simulink model "BMS_Software_NXP_Rolo"  (R2020a)
settings: Solver=FixedStepDiscrete  StartTime=0.0  StopTime=10.0  FixedStep=0.05  RelTol=1e-3  EnableMultiTasking=on
InitFcn:
  | mbd_s32k_consistency_checks(bdroot(gcs));
undefined symbols (not defined in the file or in its folder): LQFP
libraries: mbd_bcc_ec_toolbox x51, mbd_s32k1xx_ec_toolbox x16
(part 2 of 3)

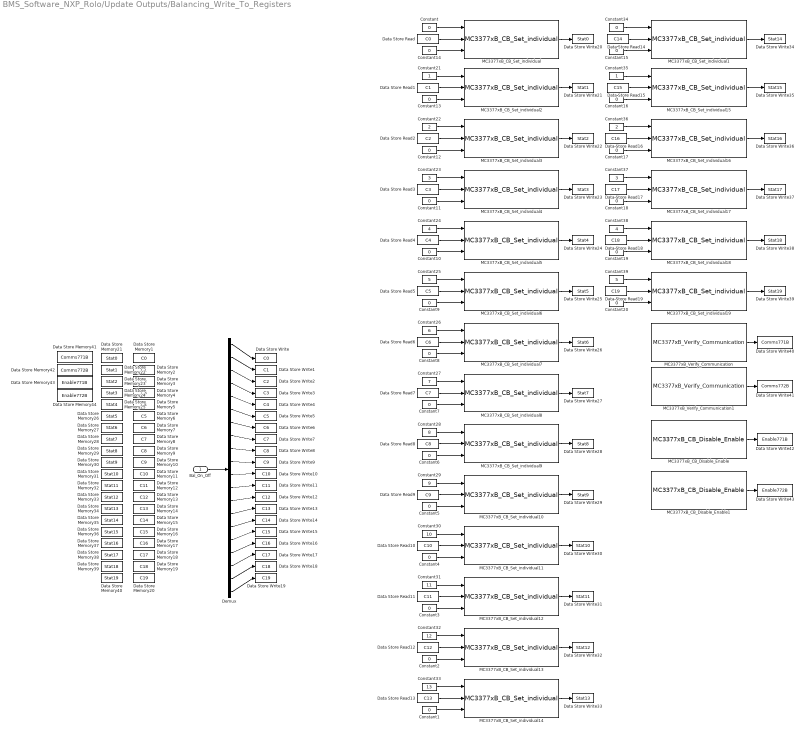
== system BMS_Software_NXP_Rolo/Update Outputs/Balancing_Write_To_Registers ==
  Bal_On_Off : Inport
  Constant : Constant  Value=0  OutDataTypeStr=uint8
  Constant{1..20} (20 alike) : Constant  Value=0  OutDataTypeStr=uint16
  Constant21 : Constant  OutDataTypeStr=uint8
  Constant22 : Constant  Value=2  OutDataTypeStr=uint8
  Constant23 : Constant  Value=3  OutDataTypeStr=uint8
  Constant24 : Constant  Value=4  OutDataTypeStr=uint8
  Constant25 : Constant  Value=5  OutDataTypeStr=uint8
  Constant26 : Constant  Value=6  OutDataTypeStr=uint8
  Constant27 : Constant  Value=7  OutDataTypeStr=uint8
  Constant28 : Constant  Value=8  OutDataTypeStr=uint8
  Constant29 : Constant  Value=9  OutDataTypeStr=uint8
  Constant30 : Constant  Value=10  OutDataTypeStr=uint8
  Constant31 : Constant  Value=11  OutDataTypeStr=uint8
  Constant32 : Constant  Value=12  OutDataTypeStr=uint8
  Constant33 : Constant  Value=13  OutDataTypeStr=uint8
  Constant34 : Constant  Value=0  OutDataTypeStr=uint8
  Constant35 : Constant  OutDataTypeStr=uint8
  Constant36 : Constant  Value=2  OutDataTypeStr=uint8
  Constant37 : Constant  Value=3  OutDataTypeStr=uint8
  Constant38 : Constant  Value=4  OutDataTypeStr=uint8
  Constant39 : Constant  Value=5  OutDataTypeStr=uint8
  Data Store Memory1 : DataStoreMemory  DataStoreName=C0  ReadBeforeWriteMsg=warning  WriteAfterWriteMsg=warning  WriteAfterReadMsg=warning  ShowAdditionalParam=off  OutDataTypeStr=boolean
  Data Store Memory10 : DataStoreMemory  DataStoreName=C9  ReadBeforeWriteMsg=warning  WriteAfterWriteMsg=warning  WriteAfterReadMsg=warning  ShowAdditionalParam=off  OutDataTypeStr=boolean
  Data Store Memory11 : DataStoreMemory  DataStoreName=C10  ReadBeforeWriteMsg=warning  WriteAfterWriteMsg=warning  WriteAfterReadMsg=warning  ShowAdditionalParam=off  OutDataTypeStr=boolean
  Data Store Memory12 : DataStoreMemory  DataStoreName=C11  ReadBeforeWriteMsg=warning  WriteAfterWriteMsg=warning  WriteAfterReadMsg=warning  ShowAdditionalParam=off  OutDataTypeStr=boolean
  Data Store Memory13 : DataStoreMemory  DataStoreName=C12  ReadBeforeWriteMsg=warning  WriteAfterWriteMsg=warning  WriteAfterReadMsg=warning  ShowAdditionalParam=off  OutDataTypeStr=boolean
  Data Store Memory14 : DataStoreMemory  DataStoreName=C13  ReadBeforeWriteMsg=warning  WriteAfterWriteMsg=warning  WriteAfterReadMsg=warning  ShowAdditionalParam=off  OutDataTypeStr=boolean
  Data Store Memory15 : DataStoreMemory  DataStoreName=C14  ReadBeforeWriteMsg=warning  WriteAfterWriteMsg=warning  WriteAfterReadMsg=warning  ShowAdditionalParam=off  OutDataTypeStr=boolean
  Data Store Memory16 : DataStoreMemory  DataStoreName=C15  ReadBeforeWriteMsg=warning  WriteAfterWriteMsg=warning  WriteAfterReadMsg=warning  ShowAdditionalParam=off  OutDataTypeStr=boolean
  Data Store Memory17 : DataStoreMemory  DataStoreName=C16  ReadBeforeWriteMsg=warning  WriteAfterWriteMsg=warning  WriteAfterReadMsg=warning  ShowAdditionalParam=off  OutDataTypeStr=boolean
  Data Store Memory18 : DataStoreMemory  DataStoreName=C17  ReadBeforeWriteMsg=warning  WriteAfterWriteMsg=warning  WriteAfterReadMsg=warning  ShowAdditionalParam=off  OutDataTypeStr=boolean
  Data Store Memory19 : DataStoreMemory  DataStoreName=C18  ReadBeforeWriteMsg=warning  WriteAfterWriteMsg=warning  WriteAfterReadMsg=warning  ShowAdditionalParam=off  OutDataTypeStr=boolean
  Data Store Memory2 : DataStoreMemory  DataStoreName=C1  ReadBeforeWriteMsg=warning  WriteAfterWriteMsg=warning  WriteAfterReadMsg=warning  ShowAdditionalParam=off  OutDataTypeStr=boolean
  Data Store Memory20 : DataStoreMemory  DataStoreName=C19  ReadBeforeWriteMsg=warning  WriteAfterWriteMsg=warning  WriteAfterReadMsg=warning  ShowAdditionalParam=off  OutDataTypeStr=boolean
  Data Store Memory21 : DataStoreMemory  DataStoreName=Stat0  ReadBeforeWriteMsg=warning  WriteAfterWriteMsg=warning  WriteAfterReadMsg=warning  ShowAdditionalParam=off  OutDataTypeStr=uint8
  Data Store Memory22 : DataStoreMemory  DataStoreName=Stat1  ReadBeforeWriteMsg=warning  WriteAfterWriteMsg=warning  WriteAfterReadMsg=warning  ShowAdditionalParam=off  OutDataTypeStr=uint8
  Data Store Memory23 : DataStoreMemory  DataStoreName=Stat2  ReadBeforeWriteMsg=warning  WriteAfterWriteMsg=warning  WriteAfterReadMsg=warning  ShowAdditionalParam=off  OutDataTypeStr=uint8
  Data Store Memory24 : DataStoreMemory  DataStoreName=Stat3  ReadBeforeWriteMsg=warning  WriteAfterWriteMsg=warning  WriteAfterReadMsg=warning  ShowAdditionalParam=off  OutDataTypeStr=uint8
  Data Store Memory25 : DataStoreMemory  DataStoreName=Stat4  ReadBeforeWriteMsg=warning  WriteAfterWriteMsg=warning  WriteAfterReadMsg=warning  ShowAdditionalParam=off  OutDataTypeStr=uint8
  Data Store Memory26 : DataStoreMemory  DataStoreName=Stat5  ReadBeforeWriteMsg=warning  WriteAfterWriteMsg=warning  WriteAfterReadMsg=warning  ShowAdditionalParam=off  OutDataTypeStr=uint8
  Data Store Memory27 : DataStoreMemory  DataStoreName=Stat6  ReadBeforeWriteMsg=warning  WriteAfterWriteMsg=warning  WriteAfterReadMsg=warning  ShowAdditionalParam=off  OutDataTypeStr=uint8
  Data Store Memory28 : DataStoreMemory  DataStoreName=Stat7  ReadBeforeWriteMsg=warning  WriteAfterWriteMsg=warning  WriteAfterReadMsg=warning  ShowAdditionalParam=off  OutDataTypeStr=uint8
  Data Store Memory29 : DataStoreMemory  DataStoreName=Stat8  ReadBeforeWriteMsg=warning  WriteAfterWriteMsg=warning  WriteAfterReadMsg=warning  ShowAdditionalParam=off  OutDataTypeStr=uint8
  Data Store Memory3 : DataStoreMemory  DataStoreName=C2  ReadBeforeWriteMsg=warning  WriteAfterWriteMsg=warning  WriteAfterReadMsg=warning  ShowAdditionalParam=off  OutDataTypeStr=boolean
  Data Store Memory30 : DataStoreMemory  DataStoreName=Stat9  ReadBeforeWriteMsg=warning  WriteAfterWriteMsg=warning  WriteAfterReadMsg=warning  ShowAdditionalParam=off  OutDataTypeStr=uint8
  Data Store Memory31 : DataStoreMemory  DataStoreName=Stat10  ReadBeforeWriteMsg=warning  WriteAfterWriteMsg=warning  WriteAfterReadMsg=warning  ShowAdditionalParam=off  OutDataTypeStr=uint8
  Data Store Memory32 : DataStoreMemory  DataStoreName=Stat11  ReadBeforeWriteMsg=warning  WriteAfterWriteMsg=warning  WriteAfterReadMsg=warning  ShowAdditionalParam=off  OutDataTypeStr=uint8
  Data Store Memory33 : DataStoreMemory  DataStoreName=Stat12  ReadBeforeWriteMsg=warning  WriteAfterWriteMsg=warning  WriteAfterReadMsg=warning  ShowAdditionalParam=off  OutDataTypeStr=uint8
  Data Store Memory34 : DataStoreMemory  DataStoreName=Stat13  ReadBeforeWriteMsg=warning  WriteAfterWriteMsg=warning  WriteAfterReadMsg=warning  ShowAdditionalParam=off  OutDataTypeStr=uint8
  Data Store Memory35 : DataStoreMemory  DataStoreName=Stat14  ReadBeforeWriteMsg=warning  WriteAfterWriteMsg=warning  WriteAfterReadMsg=warning  ShowAdditionalParam=off  OutDataTypeStr=uint8
  Data Store Memory36 : DataStoreMemory  DataStoreName=Stat15  ReadBeforeWriteMsg=warning  WriteAfterWriteMsg=warning  WriteAfterReadMsg=warning  ShowAdditionalParam=off  OutDataTypeStr=uint8
  Data Store Memory37 : DataStoreMemory  DataStoreName=Stat16  ReadBeforeWriteMsg=warning  WriteAfterWriteMsg=warning  WriteAfterReadMsg=warning  ShowAdditionalParam=off  OutDataTypeStr=uint8
  Data Store Memory38 : DataStoreMemory  DataStoreName=Stat17  ReadBeforeWriteMsg=warning  WriteAfterWriteMsg=warning  WriteAfterReadMsg=warning  ShowAdditionalParam=off  OutDataTypeStr=uint8
  Data Store Memory39 : DataStoreMemory  DataStoreName=Stat18  ReadBeforeWriteMsg=warning  WriteAfterWriteMsg=warning  WriteAfterReadMsg=warning  ShowAdditionalParam=off  OutDataTypeStr=uint8
  Data Store Memory4 : DataStoreMemory  DataStoreName=C3  ReadBeforeWriteMsg=warning  WriteAfterWriteMsg=warning  WriteAfterReadMsg=warning  ShowAdditionalParam=off  OutDataTypeStr=boolean
  Data Store Memory40 : DataStoreMemory  DataStoreName=Stat19  ReadBeforeWriteMsg=warning  WriteAfterWriteMsg=warning  WriteAfterReadMsg=warning  ShowAdditionalParam=off  OutDataTypeStr=uint8
  Data Store Memory41 : DataStoreMemory  DataStoreName=Comms771B  ReadBeforeWriteMsg=warning  WriteAfterWriteMsg=warning  WriteAfterReadMsg=warning  ShowAdditionalParam=off  OutDataTypeStr=uint8
  Data Store Memory42 : DataStoreMemory  DataStoreName=Comms772B  ReadBeforeWriteMsg=warning  WriteAfterWriteMsg=warning  WriteAfterReadMsg=warning  ShowAdditionalParam=off  OutDataTypeStr=uint8
  Data Store Memory43 : DataStoreMemory  DataStoreName=Enable771B  ReadBeforeWriteMsg=warning  WriteAfterWriteMsg=warning  WriteAfterReadMsg=warning  ShowAdditionalParam=off  OutDataTypeStr=uint8
  Data Store Memory44 : DataStoreMemory  DataStoreName=Enable772B  ReadBeforeWriteMsg=warning  WriteAfterWriteMsg=warning  WriteAfterReadMsg=warning  ShowAdditionalParam=off  OutDataTypeStr=uint8
  Data Store Memory5 : DataStoreMemory  DataStoreName=C4  ReadBeforeWriteMsg=warning  WriteAfterWriteMsg=warning  WriteAfterReadMsg=warning  ShowAdditionalParam=off  OutDataTypeStr=boolean
  Data Store Memory6 : DataStoreMemory  DataStoreName=C5  ReadBeforeWriteMsg=warning  WriteAfterWriteMsg=warning  WriteAfterReadMsg=warning  ShowAdditionalParam=off  OutDataTypeStr=boolean
  Data Store Memory7 : DataStoreMemory  DataStoreName=C6  ReadBeforeWriteMsg=warning  WriteAfterWriteMsg=warning  WriteAfterReadMsg=warning  ShowAdditionalParam=off  OutDataTypeStr=boolean
  Data Store Memory8 : DataStoreMemory  DataStoreName=C7  ReadBeforeWriteMsg=warning  WriteAfterWriteMsg=warning  WriteAfterReadMsg=warning  ShowAdditionalParam=off  OutDataTypeStr=boolean
  Data Store Memory9 : DataStoreMemory  DataStoreName=C8  ReadBeforeWriteMsg=warning  WriteAfterWriteMsg=warning  WriteAfterReadMsg=warning  ShowAdditionalParam=off  OutDataTypeStr=boolean
  Data Store Read : DataStoreRead  DataStoreName=C0
  Data Store Read1 : DataStoreRead  DataStoreName=C1
  Data Store Read10 : DataStoreRead  DataStoreName=C10
  Data Store Read11 : DataStoreRead  DataStoreName=C11
  Data Store Read12 : DataStoreRead  DataStoreName=C12
  Data Store Read13 : DataStoreRead  DataStoreName=C13
  Data Store Read14 : DataStoreRead  DataStoreName=C14
  Data Store Read15 : DataStoreRead  DataStoreName=C15
  Data Store Read16 : DataStoreRead  DataStoreName=C16
  Data Store Read17 : DataStoreRead  DataStoreName=C17
  Data Store Read18 : DataStoreRead  DataStoreName=C18
  Data Store Read19 : DataStoreRead  DataStoreName=C19
  Data Store Read2 : DataStoreRead  DataStoreName=C2
  Data Store Read3 : DataStoreRead  DataStoreName=C3
  Data Store Read4 : DataStoreRead  DataStoreName=C4
  Data Store Read5 : DataStoreRead  DataStoreName=C5
  Data Store Read6 : DataStoreRead  DataStoreName=C6
  Data Store Read7 : DataStoreRead  DataStoreName=C7
  Data Store Read8 : DataStoreRead  DataStoreName=C8
  Data Store Read9 : DataStoreRead  DataStoreName=C9
  Data Store Write : DataStoreWrite  DataStoreName=C0
  Data Store Write1 : DataStoreWrite  DataStoreName=C1
  Data Store Write10 : DataStoreWrite  DataStoreName=C10
  Data Store Write11 : DataStoreWrite  DataStoreName=C11
  Data Store Write12 : DataStoreWrite  DataStoreName=C12
  Data Store Write13 : DataStoreWrite  DataStoreName=C13
  Data Store Write14 : DataStoreWrite  DataStoreName=C14
  Data Store Write15 : DataStoreWrite  DataStoreName=C15
  Data Store Write16 : DataStoreWrite  DataStoreName=C16
  Data Store Write17 : DataStoreWrite  DataStoreName=C17
  Data Store Write18 : DataStoreWrite  DataStoreName=C18
  Data Store Write19 : DataStoreWrite  DataStoreName=C19
  Data Store Write2 : DataStoreWrite  DataStoreName=C2
  Data Store Write20 : DataStoreWrite  DataStoreName=Stat0
  Data Store Write21 : DataStoreWrite  DataStoreName=Stat1
  Data Store Write22 : DataStoreWrite  DataStoreName=Stat2
  Data Store Write23 : DataStoreWrite  DataStoreName=Stat3
  Data Store Write24 : DataStoreWrite  DataStoreName=Stat4
  Data Store Write25 : DataStoreWrite  DataStoreName=Stat5
  Data Store Write26 : DataStoreWrite  DataStoreName=Stat6
  Data Store Write27 : DataStoreWrite  DataStoreName=Stat7
  Data Store Write28 : DataStoreWrite  DataStoreName=Stat8
  Data Store Write29 : DataStoreWrite  DataStoreName=Stat9
  Data Store Write3 : DataStoreWrite  DataStoreName=C3
  Data Store Write30 : DataStoreWrite  DataStoreName=Stat10
  Data Store Write31 : DataStoreWrite  DataStoreName=Stat11
  Data Store Write32 : DataStoreWrite  DataStoreName=Stat12
  Data Store Write33 : DataStoreWrite  DataStoreName=Stat13
  Data Store Write34 : DataStoreWrite  DataStoreName=Stat14
  Data Store Write35 : DataStoreWrite  DataStoreName=Stat15
  Data Store Write36 : DataStoreWrite  DataStoreName=Stat16
  Data Store Write37 : DataStoreWrite  DataStoreName=Stat17
  Data Store Write38 : DataStoreWrite  DataStoreName=Stat18
  Data Store Write39 : DataStoreWrite  DataStoreName=Stat19
  Data Store Write4 : DataStoreWrite  DataStoreName=C4
  Data Store Write40 : DataStoreWrite  DataStoreName=Comms771B
  Data Store Write41 : DataStoreWrite  DataStoreName=Comms772B
  Data Store Write42 : DataStoreWrite  DataStoreName=Enable771B
  Data Store Write43 : DataStoreWrite  DataStoreName=Enable772B
  Data Store Write5 : DataStoreWrite  DataStoreName=C5
  Data Store Write6 : DataStoreWrite  DataStoreName=C6
  Data Store Write7 : DataStoreWrite  DataStoreName=C7
  Data Store Write8 : DataStoreWrite  DataStoreName=C8
  Data Store Write9 : DataStoreWrite  DataStoreName=C9
  Demux : Demux  Outputs=20
  MC3377xB_CB_Disable_Enable : mbd_bcc_ec_toolbox/BMS/MC3377xB_CB_Disable_Enable  bccInstance=0  bccCID=1  bccAction=Enable
  MC3377xB_CB_Disable_Enable1 : mbd_bcc_ec_toolbox/BMS/MC3377xB_CB_Disable_Enable  bccInstance=0  bccCID=2  bccAction=Enable
  MC3377xB_CB_Set_individual{,2..14} (14 alike) : mbd_bcc_ec_toolbox/BMS/MC3377xB_CB_Set_individual  bccInstance=0  bccCID=1
  MC3377xB_CB_Set_individual{1,15..19} (6 alike) : mbd_bcc_ec_toolbox/BMS/MC3377xB_CB_Set_individual  bccInstance=0  bccCID=2
  MC3377xB_Verify_Communication : mbd_bcc_ec_toolbox/BMS/MC3377xB_Verify_Communication  bccInstance=0  bccCID=1
  MC3377xB_Verify_Communication1 : mbd_bcc_ec_toolbox/BMS/MC3377xB_Verify_Communication  bccInstance=0  bccCID=2
  wires:
  Bal_On_Off/1 -> Demux/1
  Demux/1 -> Data Store Write/1
  Demux/2 -> Data Store Write1/1
  Demux/3 -> Data Store Write2/1
  Demux/4 -> Data Store Write3/1
  Demux/5 -> Data Store Write4/1
  Demux/6 -> Data Store Write5/1
  Demux/7 -> Data Store Write6/1
  Demux/8 -> Data Store Write7/1
  Demux/9 -> Data Store Write8/1
  Demux/10 -> Data Store Write9/1
  Demux/11 -> Data Store Write10/1
  Demux/12 -> Data Store Write11/1
  Demux/13 -> Data Store Write12/1
  Demux/14 -> Data Store Write13/1
  Demux/15 -> Data Store Write14/1
  Demux/16 -> Data Store Write15/1
  Demux/17 -> Data Store Write16/1
  Demux/18 -> Data Store Write17/1
  Demux/19 -> Data Store Write18/1
  Demux/20 -> Data Store Write19/1
  Data Store Read14/1 -> MC3377xB_CB_Set_individual1/2
  Data Store Read15/1 -> MC3377xB_CB_Set_individual15/2
  Data Store Read16/1 -> MC3377xB_CB_Set_individual16/2
  Data Store Read17/1 -> MC3377xB_CB_Set_individual17/2
  Data Store Read18/1 -> MC3377xB_CB_Set_individual18/2
  Data Store Read19/1 -> MC3377xB_CB_Set_individual19/2
  Data Store Read/1 -> MC3377xB_CB_Set_individual/2
  Data Store Read1/1 -> MC3377xB_CB_Set_individual2/2
  Data Store Read2/1 -> MC3377xB_CB_Set_individual3/2
  Data Store Read3/1 -> MC3377xB_CB_Set_individual4/2
  Data Store Read4/1 -> MC3377xB_CB_Set_individual5/2
  Data Store Read5/1 -> MC3377xB_CB_Set_individual6/2
  Data Store Read6/1 -> MC3377xB_CB_Set_individual7/2
  Data Store Read7/1 -> MC3377xB_CB_Set_individual8/2
  Data Store Read8/1 -> MC3377xB_CB_Set_individual9/2
  Data Store Read9/1 -> MC3377xB_CB_Set_individual10/2
  Data Store Read10/1 -> MC3377xB_CB_Set_individual11/2
  Data Store Read11/1 -> MC3377xB_CB_Set_individual12/2
  Data Store Read12/1 -> MC3377xB_CB_Set_individual13/2
  Data Store Read13/1 -> MC3377xB_CB_Set_individual14/2
  Constant1/1 -> MC3377xB_CB_Set_individual14/3
  Constant2/1 -> MC3377xB_CB_Set_individual13/3
  Constant3/1 -> MC3377xB_CB_Set_individual12/3
  Constant4/1 -> MC3377xB_CB_Set_individual11/3
  Constant5/1 -> MC3377xB_CB_Set_individual10/3
  Constant6/1 -> MC3377xB_CB_Set_individual9/3
  Constant7/1 -> MC3377xB_CB_Set_individual8/3
  Constant8/1 -> MC3377xB_CB_Set_individual7/3
  Constant9/1 -> MC3377xB_CB_Set_individual6/3
  Constant10/1 -> MC3377xB_CB_Set_individual5/3
  Constant11/1 -> MC3377xB_CB_Set_individual4/3
  Constant12/1 -> MC3377xB_CB_Set_individual3/3
  Constant13/1 -> MC3377xB_CB_Set_individual2/3
  Constant14/1 -> MC3377xB_CB_Set_individual/3
  Constant15/1 -> MC3377xB_CB_Set_individual1/3
  Constant16/1 -> MC3377xB_CB_Set_individual15/3
  Constant17/1 -> MC3377xB_CB_Set_individual16/3
  Constant18/1 -> MC3377xB_CB_Set_individual17/3
  Constant19/1 -> MC3377xB_CB_Set_individual18/3
  Constant20/1 -> MC3377xB_CB_Set_individual19/3
  Constant/1 -> MC3377xB_CB_Set_individual/1
  Constant21/1 -> MC3377xB_CB_Set_individual2/1
  Constant22/1 -> MC3377xB_CB_Set_individual3/1
  Constant23/1 -> MC3377xB_CB_Set_individual4/1
  Constant24/1 -> MC3377xB_CB_Set_individual5/1
  Constant25/1 -> MC3377xB_CB_Set_individual6/1
  Constant26/1 -> MC3377xB_CB_Set_individual7/1
  Constant27/1 -> MC3377xB_CB_Set_individual8/1
  Constant28/1 -> MC3377xB_CB_Set_individual9/1
  Constant29/1 -> MC3377xB_CB_Set_individual10/1
  Constant30/1 -> MC3377xB_CB_Set_individual11/1
  Constant31/1 -> MC3377xB_CB_Set_individual12/1
  Constant32/1 -> MC3377xB_CB_Set_individual13/1
  Constant33/1 -> MC3377xB_CB_Set_individual14/1
  Constant34/1 -> MC3377xB_CB_Set_individual1/1
  Constant35/1 -> MC3377xB_CB_Set_individual15/1
  Constant36/1 -> MC3377xB_CB_Set_individual16/1
  Constant37/1 -> MC3377xB_CB_Set_individual17/1
  Constant38/1 -> MC3377xB_CB_Set_individual18/1
  Constant39/1 -> MC3377xB_CB_Set_individual19/1
  MC3377xB_CB_Set_individual/1 -> Data Store Write20/1
  MC3377xB_CB_Set_individual2/1 -> Data Store Write21/1
  MC3377xB_CB_Set_individual3/1 -> Data Store Write22/1
  MC3377xB_CB_Set_individual4/1 -> Data Store Write23/1
  MC3377xB_CB_Set_individual5/1 -> Data Store Write24/1
  MC3377xB_CB_Set_individual6/1 -> Data Store Write25/1
  MC3377xB_CB_Set_individual7/1 -> Data Store Write26/1
  MC3377xB_CB_Set_individual8/1 -> Data Store Write27/1
  MC3377xB_CB_Set_individual9/1 -> Data Store Write28/1
  MC3377xB_CB_Set_individual10/1 -> Data Store Write29/1
  MC3377xB_CB_Set_individual11/1 -> Data Store Write30/1
  MC3377xB_CB_Set_individual12/1 -> Data Store Write31/1
  MC3377xB_CB_Set_individual13/1 -> Data Store Write32/1
  MC3377xB_CB_Set_individual14/1 -> Data Store Write33/1
  MC3377xB_CB_Set_individual1/1 -> Data Store Write34/1
  MC3377xB_CB_Set_individual15/1 -> Data Store Write35/1
  MC3377xB_CB_Set_individual16/1 -> Data Store Write36/1
  MC3377xB_CB_Set_individual17/1 -> Data Store Write37/1
  MC3377xB_CB_Set_individual18/1 -> Data Store Write38/1
  MC3377xB_CB_Set_individual19/1 -> Data Store Write39/1
  MC3377xB_Verify_Communication/1 -> Data Store Write40/1
  MC3377xB_Verify_Communication1/1 -> Data Store Write41/1
  MC3377xB_CB_Disable_Enable/1 -> Data Store Write42/1
  MC3377xB_CB_Disable_Enable1/1 -> Data Store Write43/1

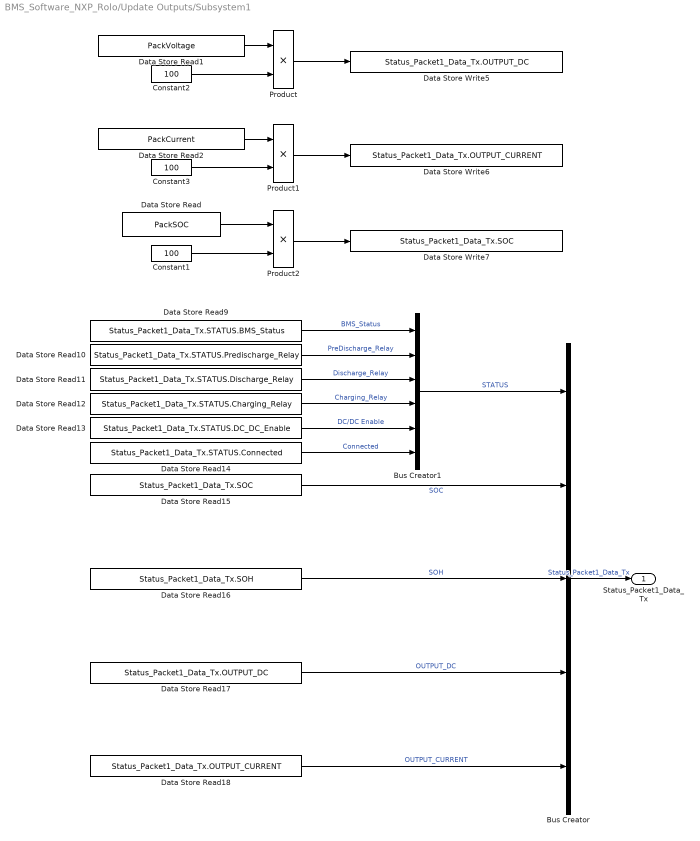
== system BMS_Software_NXP_Rolo/Update Outputs/Subsystem1 ==
  Bus Creator : BusCreator  Inputs=5  OutDataTypeStr=Bus: Status_Packet1_Data_Tx  NonVirtualBus=on
  Bus Creator1 : BusCreator  Inputs=6  OutDataTypeStr=Bus: STATUS  NonVirtualBus=on
  Constant1 : Constant  Value=100  OutDataTypeStr=single
  Constant2 : Constant  Value=100  OutDataTypeStr=single
  Constant3 : Constant  Value=100  OutDataTypeStr=single
  Data Store Read : DataStoreRead  DataStoreName=PackSOC
  Data Store Read1 : DataStoreRead  DataStoreName=PackVoltage
  Data Store Read10 : DataStoreRead  DataStoreName=Status_Packet1_Data_Tx  DataStoreElements=Status_Packet1_Data_Tx.STATUS.Predischarge_Relay
  Data Store Read11 : DataStoreRead  DataStoreName=Status_Packet1_Data_Tx  DataStoreElements=Status_Packet1_Data_Tx.STATUS.Discharge_Relay
  Data Store Read12 : DataStoreRead  DataStoreName=Status_Packet1_Data_Tx  DataStoreElements=Status_Packet1_Data_Tx.STATUS.Charging_Relay
  Data Store Read13 : DataStoreRead  DataStoreName=Status_Packet1_Data_Tx  DataStoreElements=Status_Packet1_Data_Tx.STATUS.DC_DC_Enable
  Data Store Read14 : DataStoreRead  DataStoreName=Status_Packet1_Data_Tx  DataStoreElements=Status_Packet1_Data_Tx.STATUS.Connected
  Data Store Read15 : DataStoreRead  DataStoreName=Status_Packet1_Data_Tx  DataStoreElements=Status_Packet1_Data_Tx.SOC
  Data Store Read16 : DataStoreRead  DataStoreName=Status_Packet1_Data_Tx  DataStoreElements=Status_Packet1_Data_Tx.SOH
  Data Store Read17 : DataStoreRead  DataStoreName=Status_Packet1_Data_Tx  DataStoreElements=Status_Packet1_Data_Tx.OUTPUT_DC
  Data Store Read18 : DataStoreRead  DataStoreName=Status_Packet1_Data_Tx  DataStoreElements=Status_Packet1_Data_Tx.OUTPUT_CURRENT
  Data Store Read2 : DataStoreRead  DataStoreName=PackCurrent
  Data Store Read9 : DataStoreRead  DataStoreName=Status_Packet1_Data_Tx  DataStoreElements=Status_Packet1_Data_Tx.STATUS.BMS_Status
  Data Store Write5 : DataStoreWrite  DataStoreName=Status_Packet1_Data_Tx  DataStoreElements=Status_Packet1_Data_Tx.OUTPUT_DC
  Data Store Write6 : DataStoreWrite  DataStoreName=Status_Packet1_Data_Tx  DataStoreElements=Status_Packet1_Data_Tx.OUTPUT_CURRENT
  Data Store Write7 : DataStoreWrite  DataStoreName=Status_Packet1_Data_Tx  DataStoreElements=Status_Packet1_Data_Tx.SOC
  Product : Product  OutDataTypeStr=uint16
  Product1 : Product  OutDataTypeStr=uint16
  Product2 : Product  OutDataTypeStr=uint8
  Status_Packet1_Data_Tx : Outport  OutDataTypeStr=Bus: Status_Packet1_Data_Tx
  wires:
  Bus Creator1/1 -> Bus Creator/1  "STATUS"
  Data Store Read12/1 -> Bus Creator1/4  "Charging_Relay"
  Data Store Read9/1 -> Bus Creator1/1  "BMS_Status"
  Data Store Read14/1 -> Bus Creator1/6  "Connected"
  Data Store Read13/1 -> Bus Creator1/5  "DC/DC Enable"
  Data Store Read10/1 -> Bus Creator1/2  "PreDischarge_Relay"
  Data Store Read11/1 -> Bus Creator1/3  "Discharge_Relay"
  Bus Creator/1 -> Status_Packet1_Data_Tx/1  "Status_Packet1_Data_Tx"
  Constant2/1 -> Product/2
  Constant3/1 -> Product1/2
  Data Store Read15/1 -> Bus Creator/2  "SOC"
  Data Store Read16/1 -> Bus Creator/3  "SOH"
  Product/1 -> Data Store Write5/1
  Product1/1 -> Data Store Write6/1
  Data Store Read17/1 -> Bus Creator/4  "OUTPUT_DC"
  Data Store Read18/1 -> Bus Creator/5  "OUTPUT_CURRENT"
  Data Store Read1/1 -> Product/1
  Data Store Read2/1 -> Product1/1
  Data Store Read/1 -> Product2/1
  Constant1/1 -> Product2/2
  Product2/1 -> Data Store Write7/1

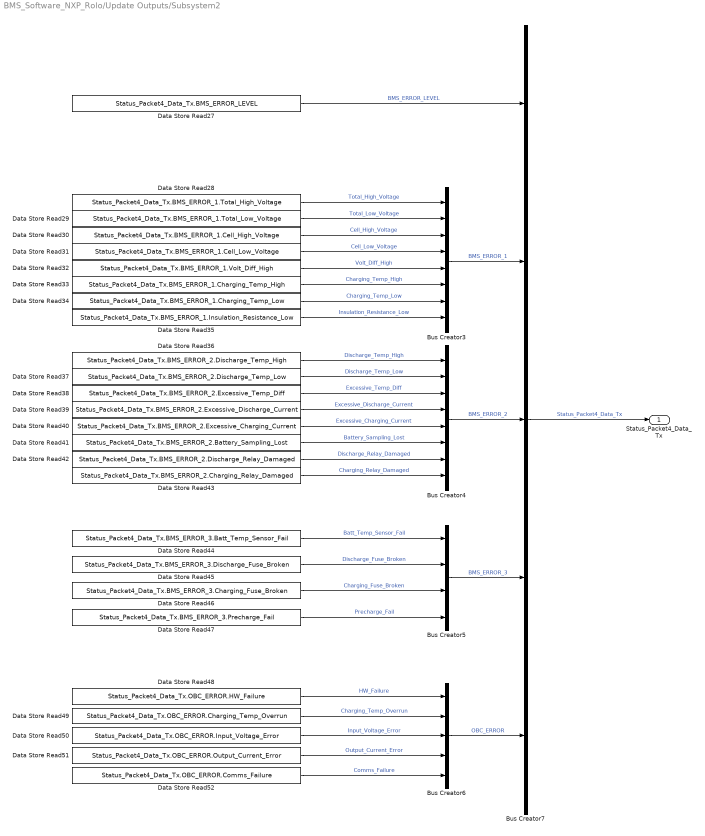
== system BMS_Software_NXP_Rolo/Update Outputs/Subsystem2 ==
  Bus Creator3 : BusCreator  Inputs=8  OutDataTypeStr=Bus: BMS_ERROR_1  NonVirtualBus=on
  Bus Creator4 : BusCreator  Inputs=8  OutDataTypeStr=Bus: BMS_ERROR_2  NonVirtualBus=on
  Bus Creator5 : BusCreator  Inputs=4  OutDataTypeStr=Bus: BMS_ERROR_3  NonVirtualBus=on
  Bus Creator6 : BusCreator  Inputs=5  OutDataTypeStr=Bus: OBC_ERROR  NonVirtualBus=on
  Bus Creator7 : BusCreator  Inputs=5  OutDataTypeStr=Bus: Status_Packet4_Data_Tx  NonVirtualBus=on
  Data Store Read27 : DataStoreRead  DataStoreName=Status_Packet4_Data_Tx  DataStoreElements=Status_Packet4_Data_Tx.BMS_ERROR_LEVEL
  Data Store Read28 : DataStoreRead  DataStoreName=Status_Packet4_Data_Tx  DataStoreElements=Status_Packet4_Data_Tx.BMS_ERROR_1.Total_High_Voltage
  Data Store Read29 : DataStoreRead  DataStoreName=Status_Packet4_Data_Tx  DataStoreElements=Status_Packet4_Data_Tx.BMS_ERROR_1.Total_Low_Voltage
  Data Store Read30 : DataStoreRead  DataStoreName=Status_Packet4_Data_Tx  DataStoreElements=Status_Packet4_Data_Tx.BMS_ERROR_1.Cell_High_Voltage
  Data Store Read31 : DataStoreRead  DataStoreName=Status_Packet4_Data_Tx  DataStoreElements=Status_Packet4_Data_Tx.BMS_ERROR_1.Cell_Low_Voltage
  Data Store Read32 : DataStoreRead  DataStoreName=Status_Packet4_Data_Tx  DataStoreElements=Status_Packet4_Data_Tx.BMS_ERROR_1.Volt_Diff_High
  Data Store Read33 : DataStoreRead  DataStoreName=Status_Packet4_Data_Tx  DataStoreElements=Status_Packet4_Data_Tx.BMS_ERROR_1.Charging_Temp_High
  Data Store Read34 : DataStoreRead  DataStoreName=Status_Packet4_Data_Tx  DataStoreElements=Status_Packet4_Data_Tx.BMS_ERROR_1.Charging_Temp_Low
  Data Store Read35 : DataStoreRead  DataStoreName=Status_Packet4_Data_Tx  DataStoreElements=Status_Packet4_Data_Tx.BMS_ERROR_1.Insulation_Resistance_Low
  Data Store Read36 : DataStoreRead  DataStoreName=Status_Packet4_Data_Tx  DataStoreElements=Status_Packet4_Data_Tx.BMS_ERROR_2.Discharge_Temp_High
  Data Store Read37 : DataStoreRead  DataStoreName=Status_Packet4_Data_Tx  DataStoreElements=Status_Packet4_Data_Tx.BMS_ERROR_2.Discharge_Temp_Low
  Data Store Read38 : DataStoreRead  DataStoreName=Status_Packet4_Data_Tx  DataStoreElements=Status_Packet4_Data_Tx.BMS_ERROR_2.Excessive_Temp_Diff
  Data Store Read39 : DataStoreRead  DataStoreName=Status_Packet4_Data_Tx  DataStoreElements=Status_Packet4_Data_Tx.BMS_ERROR_2.Excessive_Discharge_Current
  Data Store Read40 : DataStoreRead  DataStoreName=Status_Packet4_Data_Tx  DataStoreElements=Status_Packet4_Data_Tx.BMS_ERROR_2.Excessive_Charging_Current
  Data Store Read41 : DataStoreRead  DataStoreName=Status_Packet4_Data_Tx  DataStoreElements=Status_Packet4_Data_Tx.BMS_ERROR_2.Battery_Sampling_Lost
  Data Store Read42 : DataStoreRead  DataStoreName=Status_Packet4_Data_Tx  DataStoreElements=Status_Packet4_Data_Tx.BMS_ERROR_2.Discharge_Relay_Damaged
  Data Store Read43 : DataStoreRead  DataStoreName=Status_Packet4_Data_Tx  DataStoreElements=Status_Packet4_Data_Tx.BMS_ERROR_2.Charging_Relay_Damaged
  Data Store Read44 : DataStoreRead  DataStoreName=Status_Packet4_Data_Tx  DataStoreElements=Status_Packet4_Data_Tx.BMS_ERROR_3.Batt_Temp_Sensor_Fail
  Data Store Read45 : DataStoreRead  DataStoreName=Status_Packet4_Data_Tx  DataStoreElements=Status_Packet4_Data_Tx.BMS_ERROR_3.Discharge_Fuse_Broken
  Data Store Read46 : DataStoreRead  DataStoreName=Status_Packet4_Data_Tx  DataStoreElements=Status_Packet4_Data_Tx.BMS_ERROR_3.Charging_Fuse_Broken
  Data Store Read47 : DataStoreRead  DataStoreName=Status_Packet4_Data_Tx  DataStoreElements=Status_Packet4_Data_Tx.BMS_ERROR_3.Precharge_Fail
  Data Store Read48 : DataStoreRead  DataStoreName=Status_Packet4_Data_Tx  DataStoreElements=Status_Packet4_Data_Tx.OBC_ERROR.HW_Failure
  Data Store Read49 : DataStoreRead  DataStoreName=Status_Packet4_Data_Tx  DataStoreElements=Status_Packet4_Data_Tx.OBC_ERROR.Charging_Temp_Overrun
  Data Store Read50 : DataStoreRead  DataStoreName=Status_Packet4_Data_Tx  DataStoreElements=Status_Packet4_Data_Tx.OBC_ERROR.Input_Voltage_Error
  Data Store Read51 : DataStoreRead  DataStoreName=Status_Packet4_Data_Tx  DataStoreElements=Status_Packet4_Data_Tx.OBC_ERROR.Output_Current_Error
  Data Store Read52 : DataStoreRead  DataStoreName=Status_Packet4_Data_Tx  DataStoreElements=Status_Packet4_Data_Tx.OBC_ERROR.Comms_Failure
  Status_Packet4_Data_Tx : Outport  OutDataTypeStr=Bus: Status_Packet4_Data_Tx
  wires:
  Bus Creator7/1 -> Status_Packet4_Data_Tx/1  "Status_Packet4_Data_Tx"
  Data Store Read30/1 -> Bus Creator3/3  "Cell_High_Voltage"
  Data Store Read32/1 -> Bus Creator3/5  "Volt_Diff_High"
  Data Store Read34/1 -> Bus Creator3/7  "Charging_Temp_Low"
  Data Store Read29/1 -> Bus Creator3/2  "Total_Low_Voltage"
  Data Store Read31/1 -> Bus Creator3/4  "Cell_Low_Voltage"
  Bus Creator3/1 -> Bus Creator7/2  "BMS_ERROR_1"
  Bus Creator6/1 -> Bus Creator7/5  "OBC_ERROR"
  Bus Creator4/1 -> Bus Creator7/3  "BMS_ERROR_2"
  Bus Creator5/1 -> Bus Creator7/4  "BMS_ERROR_3"
  Data Store Read47/1 -> Bus Creator5/4  "Precharge_Fail"
  Data Store Read48/1 -> Bus Creator6/1  "HW_Failure"
  Data Store Read45/1 -> Bus Creator5/2  "Discharge_Fuse_Broken"
  Data Store Read33/1 -> Bus Creator3/6  "Charging_Temp_High"
  Data Store Read51/1 -> Bus Creator6/4  "Output_Current_Error"
  Data Store Read44/1 -> Bus Creator5/1  "Batt_Temp_Sensor_Fail"
  Data Store Read49/1 -> Bus Creator6/2  "Charging_Temp_Overrun"
  Data Store Read35/1 -> Bus Creator3/8  "Insulation_Resistance_Low"
  Data Store Read50/1 -> Bus Creator6/3  "Input_Voltage_Error"
  Data Store Read46/1 -> Bus Creator5/3  "Charging_Fuse_Broken"
  Data Store Read52/1 -> Bus Creator6/5  "Comms_Failure"
  Data Store Read27/1 -> Bus Creator7/1  "BMS_ERROR_LEVEL"
  Data Store Read28/1 -> Bus Creator3/1  "Total_High_Voltage"
  Data Store Read36/1 -> Bus Creator4/1  "Discharge_Temp_High"
  Data Store Read37/1 -> Bus Creator4/2  "Discharge_Temp_Low"
  Data Store Read38/1 -> Bus Creator4/3  "Excessive_Temp_Diff"
  Data Store Read39/1 -> Bus Creator4/4  "Excessive_Discharge_Current"
  Data Store Read40/1 -> Bus Creator4/5  "Excessive_Charging_Current"
  Data Store Read41/1 -> Bus Creator4/6  "Battery_Sampling_Lost"
  Data Store Read42/1 -> Bus Creator4/7  "Discharge_Relay_Damaged"
  Data Store Read43/1 -> Bus Creator4/8  "Charging_Relay_Damaged"

== system BMS_Software_NXP_Rolo/Update Outputs/Subsystem3 ==
  Bus Creator : BusCreator  Inputs=4  OutDataTypeStr=Bus: Status_Packet2_Data_Tx  NonVirtualBus=on
  Constant : Constant  Value=150  OutDataTypeStr=uint16
  Constant2 : Constant  Value=10000  OutDataTypeStr=single
  Constant3 : Constant  Value=10000  OutDataTypeStr=single
  Data Store Read1 : DataStoreRead  DataStoreName=MaxCellVoltage
  Data Store Read2 : DataStoreRead  DataStoreName=MinCellVoltage
  Data Store Read3 : DataStoreRead  DataStoreName=Status_Packet2_Data_Tx  DataStoreElements=Status_Packet2_Data_Tx.MAX_BUS_CURRENT
  Data Store Read4 : DataStoreRead  DataStoreName=Status_Packet2_Data_Tx  DataStoreElements=Status_Packet2_Data_Tx.MAX_REGEN_CURRENT
  Data Store Read5 : DataStoreRead  DataStoreName=Status_Packet2_Data_Tx  DataStoreElements=Status_Packet2_Data_Tx.HIGHEST_CELL_VOLTAGE
  Data Store Read6 : DataStoreRead  DataStoreName=Status_Packet2_Data_Tx  DataStoreElements=Status_Packet2_Data_Tx.LOWEST_CELL_VOLTAGE
  Data Store Write : DataStoreWrite  DataStoreName=Status_Packet2_Data_Tx  DataStoreElements=Status_Packet2_Data_Tx.MAX_BUS_CURRENT
  Data Store Write1 : DataStoreWrite  DataStoreName=Status_Packet2_Data_Tx  DataStoreElements=Status_Packet2_Data_Tx.HIGHEST_CELL_VOLTAGE
  Data Store Write2 : DataStoreWrite  DataStoreName=Status_Packet2_Data_Tx  DataStoreElements=Status_Packet2_Data_Tx.LOWEST_CELL_VOLTAGE
  Product : Product  OutDataTypeStr=uint16
  Product1 : Product  OutDataTypeStr=uint16
  Status_Packet2_Data_Tx : Outport  OutDataTypeStr=Bus: Status_Packet2_Data_Tx
  wires:
  Bus Creator/1 -> Status_Packet2_Data_Tx/1  "Status_Packet2_Data_Tx"
  Data Store Read4/1 -> Bus Creator/2  "MAX_REGEN_CURRENT"
  Data Store Read1/1 -> Product/1
  Data Store Read2/1 -> Product1/1
  Constant3/1 -> Product1/2
  Constant2/1 -> Product/2
  Data Store Read5/1 -> Bus Creator/3  "HIGHEST_CELL_VOLTAGE"
  Data Store Read6/1 -> Bus Creator/4  "LOWEST_CELL_VOLTAGE"
  Data Store Read3/1 -> Bus Creator/1  "MAX_BUS_CURRENT"
  Product/1 -> Data Store Write1/1
  Product1/1 -> Data Store Write2/1
  Constant/1 -> Data Store Write/1

== system BMS_Software_NXP_Rolo/Update Outputs/Subsystem4 ==
  Add1 : Sum  Inputs=+-  OutDataTypeStr=uint8
  Add2 : Sum  Inputs=+-  OutDataTypeStr=uint8
  Bus Creator : BusCreator  Inputs=5  OutDataTypeStr=Bus: Status_Packet3_Data_Tx  NonVirtualBus=on
  Constant : Constant  Value=273.15  OutDataTypeStr=single
  Constant1 : Constant  Value=273.15  OutDataTypeStr=single
  Data Store Read1 : DataStoreRead  DataStoreName=MaxCellTemp
  Data Store Read2 : DataStoreRead  DataStoreName=MinCellTemp
  Data Store Read3 : DataStoreRead  DataStoreName=Status_Packet3_Data_Tx  DataStoreElements=Status_Packet3_Data_Tx.MAX_TEMP
  Data Store Read4 : DataStoreRead  DataStoreName=Status_Packet3_Data_Tx  DataStoreElements=Status_Packet3_Data_Tx.MAX_TEMP_NUMBER
  Data Store Read5 : DataStoreRead  DataStoreName=Status_Packet3_Data_Tx  DataStoreElements=Status_Packet3_Data_Tx.MIN_TEMP
  Data Store Read6 : DataStoreRead  DataStoreName=Status_Packet3_Data_Tx  DataStoreElements=Status_Packet3_Data_Tx.MIN_TEMP_NUMBER
  Data Store Read7 : DataStoreRead  DataStoreName=Status_Packet3_Data_Tx  DataStoreElements=Status_Packet3_Data_Tx.CHARGE_DISCHARGE_CYCLES
  Data Store Write : DataStoreWrite  DataStoreName=Status_Packet3_Data_Tx  DataStoreElements=Status_Packet3_Data_Tx.MAX_TEMP
  Data Store Write1 : DataStoreWrite  DataStoreName=Status_Packet3_Data_Tx  DataStoreElements=Status_Packet3_Data_Tx.MIN_TEMP
  Status_Packet3_Data_Tx : Outport  OutDataTypeStr=Bus: Status_Packet3_Data_Tx
  wires:
  Data Store Read4/1 -> Bus Creator/2  "MAX_TEMP_NUMBER"
  Data Store Read6/1 -> Bus Creator/4  "MIN_TEMP_NUMBER"
  Bus Creator/1 -> Status_Packet3_Data_Tx/1  "Status_Packet3_Data_Tx"
  Data Store Read7/1 -> Bus Creator/5  "CHARGE_DISCHARGE_CYCLES"
  Data Store Read1/1 -> Add2/1
  Constant/1 -> Add2/2
  Data Store Read2/1 -> Add1/1
  Constant1/1 -> Add1/2
  Add1/1 -> Data Store Write1/1  "MIN_TEMP"
  Add2/1 -> Data Store Write/1  "MAX_TEMP"
  Data Store Read3/1 -> Bus Creator/1  "MAX_TEMP"
  Data Store Read5/1 -> Bus Creator/3  "MIN_TEMP"
